simulink model "grading_system"  (R2021a)
settings: Solver=FixedStepDiscrete  StartTime=0.0  StopTime=10.0  RelTol=1e-3  EnableMultiTasking=on
settings Model: Creator=iT-User  LastModifiedBy=iT-User
settings DataIOCC: ReturnWorkspaceOutputs=off
settings OptimizationCC: DefaultParameterBehavior=Inlined  InlineInvariantSignals=on  EnableMemcpy=off  LifeSpan=1  EfficientTunableParamExpr=on
settings DebuggingCC: UnderspecifiedInitializationDetection=Classic  MergeDetectMultiDrivingBlocksExec=none  SFMachineParentedDataDiag=warning  ArithmeticOperatorsInVariantConditions=warning
settings ModelReferenceCC: PropagateSignalLabelsOutOfModel=off
settings SFSimCC: MATLABDynamicMemAlloc=off  CustomCodeUndefinedFunction=UseInterfaceOnly
settings RTWCC: SystemTargetFile=ert.tlc  GenCodeOnly=on  TemplateMakefile=ert_default_tmf  GenerateReport=on  IncludeHyperlinkInReport=on  LaunchReport=on  GenerateTraceInfo=on  GenerateTraceReport=on  GenerateTraceReportSl=on  GenerateTraceReportSf=on  GenerateTraceReportEml=on
settings CodeAppCC: ForceParamTrailComments=on  IgnoreCustomStorageClasses=off  OperatorAnnotations=on  SimulinkDataObjDesc=on  SFDataObjDesc=on  MATLABFcnDesc=on  InsertBlockDesc=on  StateflowObjectComments=on  MATLABSourceComments=on
settings ERTTargetCC: MultiwordLength=2048  GenerateSampleERTMain=on  InlinedParameterPlacement=NonHierarchical  ERTCustomFileTemplate=example_file_process.tlc

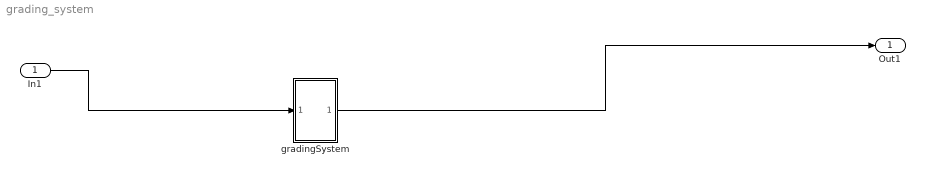
== system grading_system ==
  In1 : Inport
  gradingSystem : Subsystem
  Out1 : Outport
  wires:
  In1/1 -> gradingSystem/1(In1)
  gradingSystem/1(Out1) -> Out1/1

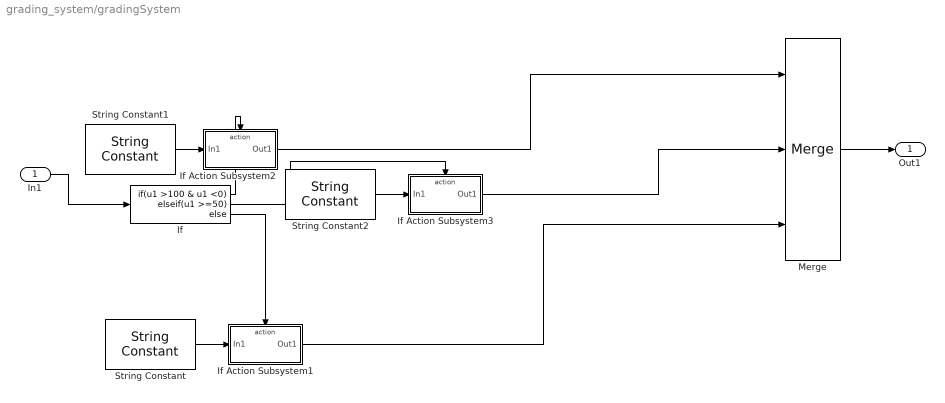
== system grading_system/gradingSystem ==
  In1 : Inport
  If : If  IfExpression=u1 >100 & u1 <0  ElseIfExpressions=u1 >=50
  If Action Subsystem1 : Subsystem  TreatAsAtomicUnit=on
  If Action Subsystem2 : Subsystem  TreatAsAtomicUnit=on
  If Action Subsystem3 : Subsystem  TreatAsAtomicUnit=on
  Merge : Merge  Inputs=3
  String Constant : StringConstant  String="\"Failed\""
  String Constant1 : StringConstant  String="\"Invalid\""
  String Constant2 : StringConstant  String="\"Passed\""
  Out1 : Outport
  wires:
  If/3 -> If Action Subsystem1/Action
  If/1 -> If Action Subsystem2/Action
  String Constant/1 -> If Action Subsystem1/1(In1)
  String Constant2/1 -> If Action Subsystem3/1(In1)
  If Action Subsystem2/1(Out1) -> Merge/1
  String Constant1/1 -> If Action Subsystem2/1(In1)
  In1/1 -> If/1
  If Action Subsystem3/1(Out1) -> Merge/2
  If Action Subsystem1/1(Out1) -> Merge/3
  If/2 -> If Action Subsystem3/Action
  Merge/1 -> Out1/1

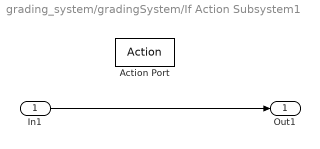
== system grading_system/gradingSystem/If Action Subsystem1 ==
  In1 : Inport
  Action Port : ActionPort  InitializeStates=reset  ActionPortLabel=else
  Out1 : Outport
  wires:
  In1/1 -> Out1/1

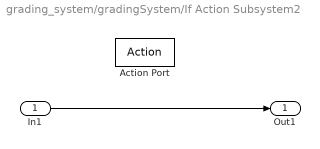
== system grading_system/gradingSystem/If Action Subsystem2 ==
  In1 : Inport
  Action Port : ActionPort  InitializeStates=reset  ActionPortLabel=if(u1 >100 & u1 <0)
  Out1 : Outport
  wires:
  In1/1 -> Out1/1

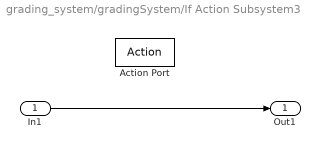
== system grading_system/gradingSystem/If Action Subsystem3 ==
  In1 : Inport
  Action Port : ActionPort  InitializeStates=reset  ActionPortLabel=elseif(u1 >=50)
  Out1 : Outport
  wires:
  In1/1 -> Out1/1
